simulink model "before_decode_out_sin_scope"  (Simulink 7.2)
settings: Solver=ode45  StartTime=0.0  StopTime=0.5  RelTol=1e-3
libraries: commutil2 x1, dspbuff3 x1, dspquant2 x1
settings Model: Creator=Administrator  LastModifiedBy=Administrator

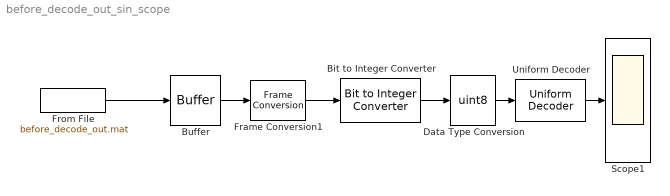
== system before_decode_out_sin_scope ==
  Bit to Integer Converter : commutil2/Bit to Integer Converter  nbits=8  bitOrder=MSB first  signedOutputValues=Unsigned  outDtype=Same as input  outDtypeSigned=Inherit via internal rule
  Buffer : dspbuff3/Buffer  N=8  V=0  ic=0
  Data Type Conversion : DataTypeConversion  OutDataTypeMode=uint8  OutDataType=sfix(16)  OutScaling=2^0  OutDataTypeStr=uint8
  Frame Conversion1 : FrameConversion  OutFrame=Sample-based
  From File : FromFile  FileName=before_decode_out.mat  SampleTime=1/1000
  Scope1 : Scope
      settings: MaxDataPoints=100000
  Uniform Decoder : dspquant2/Uniform Decoder  peak=1  bits=8  overflowMode=Saturate  otype=Double
  wires:
  Buffer/1 -> Frame Conversion1/1
  Frame Conversion1/1 -> Bit to Integer Converter/1
  Bit to Integer Converter/1 -> Data Type Conversion/1
  Data Type Conversion/1 -> Uniform Decoder/1
  Uniform Decoder/1 -> Scope1/1
  From File/1 -> Buffer/1
